simulink model "motor_ctrl_with_PID"  (R2023b)
settings: Solver=FixedStepAuto  StartTime=0.0  StopTime=inf  FixedStep=Ts  RelTol=1e-3
InitFcn:
  | params
  | pin_params
undefined symbols (not defined in the file or in its folder): den_Gd, encoder_scale, J, Kb, KD, Kf, KI, Km, KP, L, num_Gd, R, Vlim, Wref
libraries: arduinolib x12, simulink x6, arduinosensorlib x6
settings Model: SimulationMode=external  ExtModeTrigDuration=2  Creator=SJ  LastModifiedBy=tkdle
settings SolverCC: AutoInsertRateTranBlk=on
settings OptimizationCC: EnhancedBackFolding=on  PassReuseOutputArgsAs=Individual arguments  ZeroExternalMemoryAtStartup=off  ZeroInternalMemoryAtStartup=off  MaxStackSize=64  OptimizeBlockOrder=speed  DifferentSizesBufferReuse=on  OptimizationCustomize=off  EfficientTunableParamExpr=on
settings DebuggingCC: MultiTaskRateTransMsg=warning  ParameterTunabilityLossMsg=error
settings HardwareCC: ProdBitPerInt=16  ProdBitPerPointer=16  ProdBitPerSizeT=16  ProdBitPerPtrDiffT=16  ProdLargestAtomicFloat=None  ProdWordSize=8  ProdHWDeviceType=Atmel->AVR
settings SFSimCC: MATLABDynamicMemAlloc=off
settings RTWCC: Description=Embedded Coder  SystemTargetFile=ert.tlc  HardwareBoard=Arduino Mega 2560  TemplateMakefile=ert_default_tmf  Toolchain=Arduino AVR  BuildConfiguration=Faster Runs
settings CodeAppCC: ForceParamTrailComments=on  IgnoreCustomStorageClasses=off  OperatorAnnotations=on  SimulinkDataObjDesc=on  SFDataObjDesc=on  InsertBlockDesc=on
settings ERTTargetCC: SupportContinuousTime=on  SupportVariableSizeSignals=on  ExtMode=on  ExtModeTransport=3  ExtModeStaticAlloc=on  ExtModeAutomaticAllocSize=off  ExtModeStaticAllocSize=2048  ExtModeMexFile=ext_xcp  ExtModeMexArgs=0 3 921600  ExtModeIntrfLevel=Level2 - Open

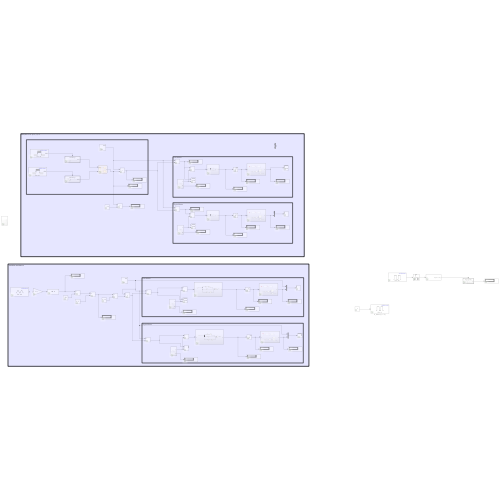
[thumbnail: Simulink's stored preview of the top-level diagram]
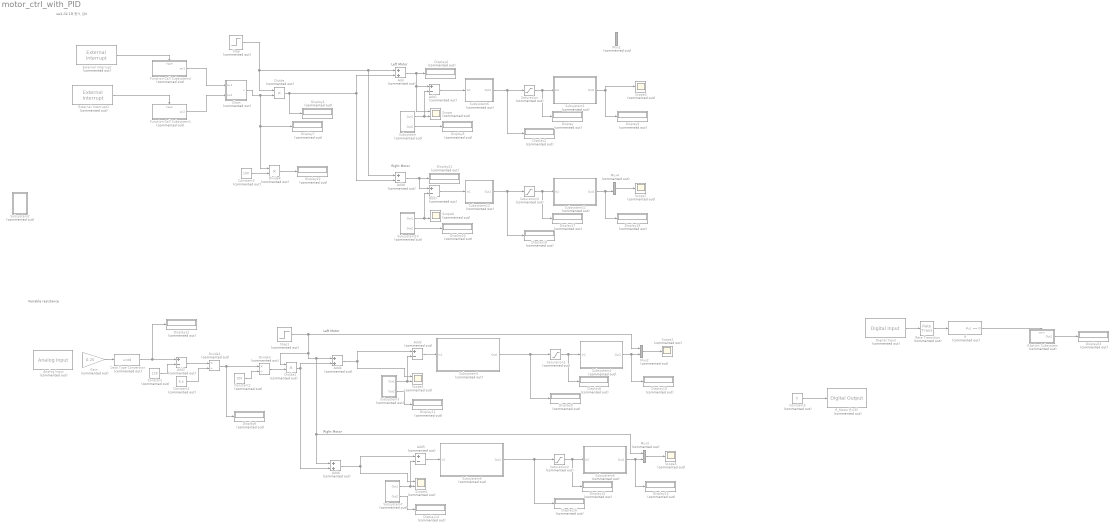
== system motor_ctrl_with_PID ==
  note: Left Motor
  note: Left Motor
  note: Right Motor
  note: Variable resistance
  note: sw1,2로 1퍼 증가, 감소
  note: Right Motor
  Add : Sum  Commented=on
  Add{1..3,5,7..8} (6 alike) : Sum  Commented=on  Inputs=+-
  Add4 : Sum  Commented=on
  Add6 : Sum  Commented=on
  Analog Input : arduinolib/Analog Input  Commented=on  pinNumber=8  ReadResultsOnly=off  ConversionTriggerSource=Software  ExternalTriggerType=uint32( 0 )  OutputDataType=uint16  EnableConversionCompleteNotify=off  EnableOuputStatus=off  SampleTime=-1  blockPlatform=arduino
  Chart : Stateflow chart  Commented=on  TreatAsAtomicUnit=on
  Constant : Constant  Commented=on  Value=128
  Constant1 : Constant  Commented=on  Value=6.4
  Constant2 : Constant  Commented=on  Value=100
  Constant3 : Constant  Commented=on  Value=100
  Constant5 : Constant  Commented=on  Value=0
  Data Type Conversion : DataTypeConversion  Commented=on  OutDataTypeStr=uint8  SaturateOnIntegerOverflow=off  RndMeth=Floor
  Digital Input : arduinolib/Digital Input  Commented=on  pinNumber=20  mode=Default  Direction=input  SampleTime=0.1  blockPlatform=arduino
  Display{,1..23} (24 alike) : Display  Commented=on
  Divide : Product  Commented=on  Inputs=**
  Divide1 : Product  Commented=on  Inputs=*/
  Divide2 : Product  Commented=on  Inputs=**
  Divide3 : Product  Commented=on  Inputs=*/
  Divide4 : Product  Commented=on  Inputs=**
  External Interrupt : arduinolib/External Interrupt  Commented=on  Pin=20  PullUp=off  Mode=FALLING  InterruptSimulationInput=off
  External Interrupt1 : arduinolib/External Interrupt  Commented=on  Pin=21  PullUp=off  Mode=FALLING  InterruptSimulationInput=off
  Function-Call Subsystem1 : Subsystem  Commented=on  TreatAsAtomicUnit=on
  Function-Call Subsystem4 : Subsystem  Commented=on  TreatAsAtomicUnit=on
  Gain : Gain  Commented=on  Gain=0.25
  If : If  Commented=on  IfExpression=u1 == 0  ShowElse=off
  If Action Subsystem : Subsystem  Commented=on  TreatAsAtomicUnit=on
  Mux{1..4} (4 alike) : Mux  Commented=on  Inputs=2
  R_Motor(반시계) : arduinolib/Digital Output  Commented=on  pinNumber=Motor_R_Direction  Direction=output  blockPlatform=arduino
  Rate Transition : RateTransition  Commented=on  OutPortSampleTime=0.5
  Saturation{,1..3} (4 alike) : Saturate  Commented=on  UpperLimit=12  LowerLimit=0
  Scope{,1,4,6} (4 alike) : Scope  Commented=on  NumInputPorts=2
  Scope{2..3,5,7} (4 alike) : Scope  Commented=on
  Step : Step  Commented=on  After=Wref  SampleTime=0
  Step1 : Step  Commented=on  After=Wref  SampleTime=0
  Subsystem : Subsystem  Commented=on
  Subsystem1 : Subsystem  Commented=on
  Subsystem10 : Subsystem  Commented=on
  Subsystem11 : Subsystem  Commented=on
  Subsystem12 : Subsystem  Commented=on
  Subsystem2 : Subsystem  Commented=on
  Subsystem3 : Subsystem  Commented=on
  Subsystem4 : Subsystem  Commented=on
  Subsystem5 : Subsystem  Commented=on
  Subsystem6 : Subsystem  Commented=on
  Subsystem7 : Subsystem  Commented=on
  Subsystem8 : Subsystem  Commented=on
  Subsystem9 : Subsystem  Commented=on
  wires:
  Subsystem/1(Out1) -> Add1/2, Scope/2
  Saturation/1 -> Subsystem1/1(In2), Display/1
  Subsystem1/1(Out1) -> Scope3/1, Display3/1
  External Interrupt/1 -> Function-Call Subsystem4/Trigger
  External Interrupt1/1 -> Function-Call Subsystem1/Trigger
  Function-Call Subsystem4/1(sw1) -> Chart/1(sw1)
  Function-Call Subsystem1/1(sw2) -> Chart/2(sw2)
  Step/1 -> Divide/1, Add8/1, Add/1
  Divide/1 -> Display1/1, Add/2, Add8/2
  Chart/1(n) -> Divide4/1, Display7/1, Divide/2
  Subsystem/2(Out2) -> Display5/1
  Gain/1 -> Data Type Conversion/1
  Step1/1 -> Mux2/1, Add6/1, Mux3/1, Add4/1, Divide2/1
  Data Type Conversion/1 -> Display12/1, Add2/1
  Constant/1 -> Add2/2
  Divide1/1 -> Display6/1, Divide3/1
  Add2/1 -> Divide1/1
  Constant1/1 -> Divide1/2
  Divide2/1 -> Add6/2, Add4/2
  Constant2/1 -> Divide3/2
  Divide3/1 -> Divide2/2
  Add/1 -> Scope/1, Add1/1, Display4/1
  Saturation1/1 -> Subsystem4/1(In2), Display8/1
  Subsystem3/2(Out2) -> Display11/1
  Subsystem3/1(Out1) -> Add3/2, Scope1/2
  Subsystem4/1(Out1) -> Display10/1, Mux2/2
  Mux2/1 -> Scope2/1
  Add4/1 -> Add3/1, Scope1/1
  Subsystem5/1(Out1) -> Display9/1, Saturation1/1
  Add3/1 -> Subsystem5/1(In1)
  Subsystem6/1(Out1) -> Display2/1, Saturation/1
  Add1/1 -> Subsystem6/1(In1)
  Add6/1 -> Add5/1, Scope4/1
  Mux3/1 -> Scope5/1
  Subsystem7/2(Out2) -> Display14/1
  Subsystem8/1(Out1) -> Display13/1, Mux3/2
  Subsystem7/1(Out1) -> Add5/2, Scope4/2
  Add5/1 -> Subsystem9/1(In1)
  Saturation2/1 -> Subsystem8/1(In2), Display15/1
  Subsystem9/1(Out1) -> Display16/1, Saturation2/1
  Add7/1 -> Subsystem12/1(In1)
  Subsystem11/1(Out1) -> Display19/1, Mux4/2
  Saturation3/1 -> Subsystem11/1(In2), Display17/1
  Mux4/1 -> Scope7/1
  Subsystem10/1(Out1) -> Add7/2, Scope6/2
  Subsystem12/1(Out1) -> Display18/1, Saturation3/1
  Subsystem10/2(Out2) -> Display20/1
  Add8/1 -> Add7/1, Display21/1
  Divide4/1 -> Display22/1
  Constant3/1 -> Divide4/2
  Digital Input/1 -> Rate Transition/1
  If/1 -> If Action Subsystem/Action
  If Action Subsystem/1(Out1) -> Display23/1
  Rate Transition/1 -> If/1
  Constant5/1 -> R_Motor(반시계)/1

== system motor_ctrl_with_PID/Function-Call Subsystem1 ==
  function : TriggerPort  TriggerType=function-call  VariantControl=(inherit)
  Add : Sum  Inputs=+-
  Constant : Constant
  Delay : Delay  DelayLength=1
  sw2 : Outport
  wires:
  Add/1 -> Delay/1, sw2/1
  Delay/1 -> Add/2
  Constant/1 -> Add/1

== system motor_ctrl_with_PID/Function-Call Subsystem4 ==
  function : TriggerPort  TriggerType=function-call  VariantControl=(inherit)
  Add : Sum  Inputs=+-
  Constant : Constant
  Delay : Delay  DelayLength=1
  sw1 : Outport
  wires:
  Add/1 -> sw1/1, Delay/1
  Delay/1 -> Add/2
  Constant/1 -> Add/1

== system motor_ctrl_with_PID/If Action Subsystem ==
  Action Port : ActionPort  ActionPortLabel=if(u1 == 0)
  Add : Sum
  Constant : Constant
  Constant1 : Constant  Value=3
  Delay : Delay  DelayLength=1
  Mod : Math  Operator=mod
  Out1 : Outport
  wires:
  Mod/1 -> Delay/1, Out1/1
  Delay/1 -> Add/2
  Constant/1 -> Add/1
  Add/1 -> Mod/1
  Constant1/1 -> Mod/2

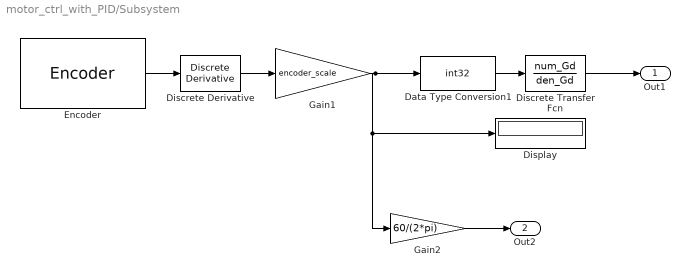
== system motor_ctrl_with_PID/Subsystem ==
  Data Type Conversion1 : DataTypeConversion  OutDataTypeStr=int32  SaturateOnIntegerOverflow=off  RndMeth=Floor
  Discrete Transfer Fcn : DiscreteTransferFcn  Numerator=num_Gd  Denominator=den_Gd
  Discrete Derivative : simulink/Discrete/Discrete Derivative  gainval=1.0  ICPrevScaledInput=0.0  OutMin=[]  OutMax=[]  OutDataType=fixdt(1, 16)  OutScaling=2^-10  DoSatur=off
  Display : Display
  Encoder : arduinosensorlib/Encoder  InputA=18  InputB=19  Mode=No reset  SampleTime=-1
  Gain1 : Gain  Gain=encoder_scale
  Gain2 : Gain  Gain=60/(2*pi)
  Out1 : Outport
  Out2 : Outport  Port=2
  wires:
  Gain1/1 -> Display/1, Gain2/1, Data Type Conversion1/1
  Encoder/1 -> Discrete Derivative/1
  Gain2/1 -> Out2/1
  Data Type Conversion1/1 -> Discrete Transfer Fcn/1
  Discrete Derivative/1 -> Gain1/1
  Discrete Transfer Fcn/1 -> Out1/1

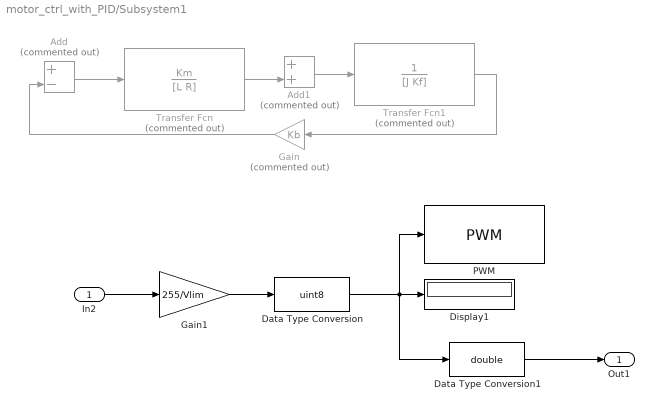
== system motor_ctrl_with_PID/Subsystem1 ==
  In2 : Inport
  Add : Sum  Commented=on  Inputs=+-
  Add1 : Sum  Commented=on
  Data Type Conversion : DataTypeConversion  OutDataTypeStr=uint8  SaturateOnIntegerOverflow=off  RndMeth=Floor
  Data Type Conversion1 : DataTypeConversion  OutDataTypeStr=double  SaturateOnIntegerOverflow=off  RndMeth=Floor
  Display1 : Display
  Gain : Gain  Commented=on  Gain=Kb
  Gain1 : Gain  Gain=255/Vlim
  PWM : arduinolib/PWM  pinNumber=11  frequencyType=Default  desiredFrequency=490.2  achievableFrequency=490.2
  Transfer Fcn : TransferFcn  Commented=on  Numerator=Km  Denominator=[L R]
  Transfer Fcn1 : TransferFcn  Commented=on  Numerator=1  Denominator=[J Kf]
  Out1 : Outport
  wires:
  ? -> Add/1
  ? -> Add1/1
  Add/1 -> Transfer Fcn/1
  Add1/1 -> Transfer Fcn1/1
  Transfer Fcn/1 -> Add1/2
  Gain/1 -> Add/2
  Transfer Fcn1/1 -> Gain/1
  In2/1 -> Gain1/1
  Gain1/1 -> Data Type Conversion/1
  Data Type Conversion1/1 -> Out1/1
  Data Type Conversion/1 -> Data Type Conversion1/1, Display1/1, PWM/1

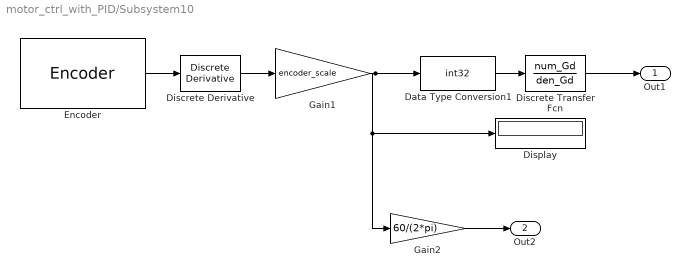
== system motor_ctrl_with_PID/Subsystem10 ==
  Data Type Conversion1 : DataTypeConversion  OutDataTypeStr=int32  SaturateOnIntegerOverflow=off  RndMeth=Floor
  Discrete Transfer Fcn : DiscreteTransferFcn  Numerator=num_Gd  Denominator=den_Gd
  Discrete Derivative : simulink/Discrete/Discrete Derivative  gainval=1.0  ICPrevScaledInput=0.0  OutMin=[]  OutMax=[]  OutDataType=fixdt(1, 16)  OutScaling=2^-10  DoSatur=off
  Display : Display
  Encoder : arduinosensorlib/Encoder  InputA=20  InputB=21  Mode=No reset  SampleTime=-1
  Gain1 : Gain  Gain=encoder_scale
  Gain2 : Gain  Gain=60/(2*pi)
  Out1 : Outport
  Out2 : Outport  Port=2
  wires:
  Gain1/1 -> Display/1, Gain2/1, Data Type Conversion1/1
  Encoder/1 -> Discrete Derivative/1
  Gain2/1 -> Out2/1
  Data Type Conversion1/1 -> Discrete Transfer Fcn/1
  Discrete Derivative/1 -> Gain1/1
  Discrete Transfer Fcn/1 -> Out1/1

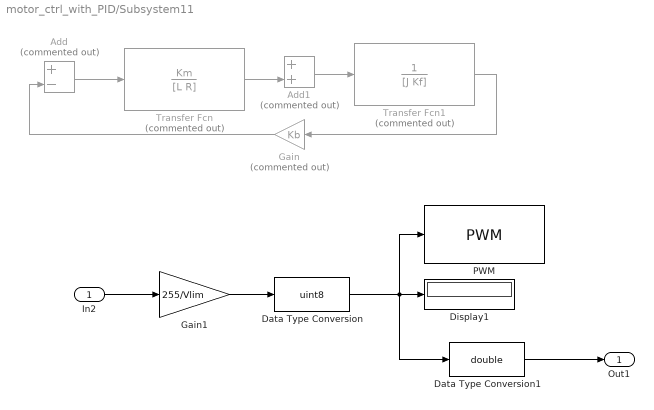
== system motor_ctrl_with_PID/Subsystem11 ==
  In2 : Inport
  Add : Sum  Commented=on  Inputs=+-
  Add1 : Sum  Commented=on
  Data Type Conversion : DataTypeConversion  OutDataTypeStr=uint8  SaturateOnIntegerOverflow=off  RndMeth=Floor
  Data Type Conversion1 : DataTypeConversion  OutDataTypeStr=double  SaturateOnIntegerOverflow=off  RndMeth=Floor
  Display1 : Display
  Gain : Gain  Commented=on  Gain=Kb
  Gain1 : Gain  Gain=255/Vlim
  PWM : arduinolib/PWM  pinNumber=11  frequencyType=Default  desiredFrequency=490.2  achievableFrequency=490.2
  Transfer Fcn : TransferFcn  Commented=on  Numerator=Km  Denominator=[L R]
  Transfer Fcn1 : TransferFcn  Commented=on  Numerator=1  Denominator=[J Kf]
  Out1 : Outport
  wires:
  ? -> Add/1
  ? -> Add1/1
  Add/1 -> Transfer Fcn/1
  Add1/1 -> Transfer Fcn1/1
  Transfer Fcn/1 -> Add1/2
  Gain/1 -> Add/2
  Transfer Fcn1/1 -> Gain/1
  In2/1 -> Gain1/1
  Gain1/1 -> Data Type Conversion/1
  Data Type Conversion1/1 -> Out1/1
  Data Type Conversion/1 -> Data Type Conversion1/1, Display1/1, PWM/1

== system motor_ctrl_with_PID/Subsystem12 ==
  In1 : Inport
  Derivative1 : Derivative  Commented=on
  Gain4 : Gain  Commented=on  Gain=KI
  Gain5 : Gain  Commented=on  Gain=KP
  Gain6 : Gain  Commented=on  Gain=KD
  Integrator1 : Integrator  Commented=on
  Subtract1 : Sum  Commented=on  Inputs=+++
  Out1 : Outport
  wires:
  Derivative1/1 -> Subtract1/3
  Gain4/1 -> Integrator1/1
  Integrator1/1 -> Subtract1/1
  Gain6/1 -> Derivative1/1
  Subtract1/1 -> Out1/1
  In1/1 -> Gain5/1, Gain6/1, Gain4/1
  Gain5/1 -> Subtract1/2

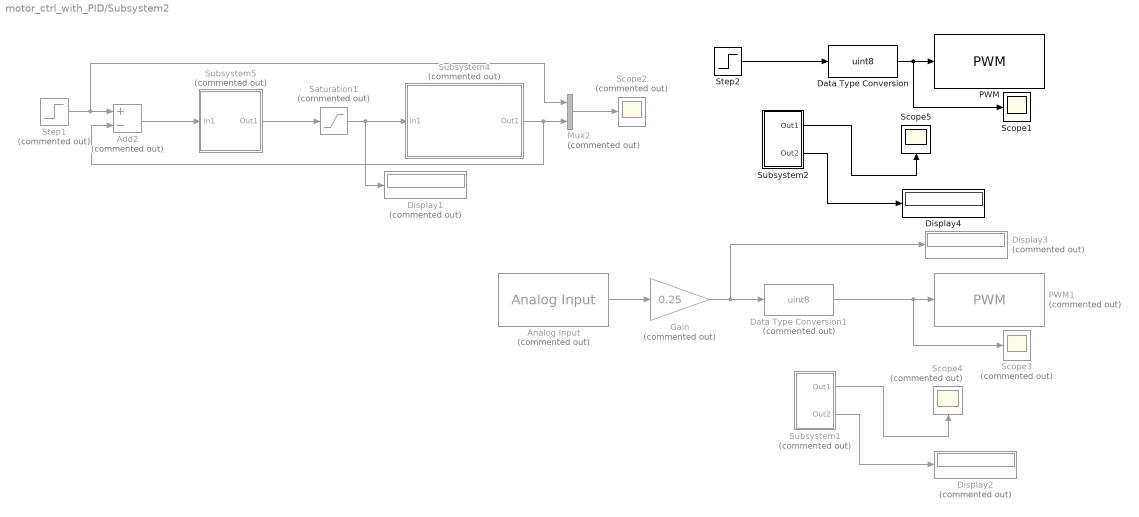
== system motor_ctrl_with_PID/Subsystem2 ==
  Add2 : Sum  Commented=on  Inputs=+-
  Analog Input : arduinolib/Analog Input  Commented=on  pinNumber=8  ReadResultsOnly=off  ConversionTriggerSource=Software  ExternalTriggerType=uint32( 0 )  OutputDataType=uint16  EnableConversionCompleteNotify=off  EnableOuputStatus=off  SampleTime=-1  blockPlatform=arduino
  Data Type Conversion : DataTypeConversion  OutDataTypeStr=uint8  SaturateOnIntegerOverflow=off  RndMeth=Floor
  Data Type Conversion1 : DataTypeConversion  Commented=on  OutDataTypeStr=uint8  SaturateOnIntegerOverflow=off  RndMeth=Floor
  Display1 : Display  Commented=on
  Display2 : Display  Commented=on
  Display3 : Display  Commented=on
  Display4 : Display
  Gain : Gain  Commented=on  Gain=0.25
  Mux2 : Mux  Commented=on  Inputs=2
  PWM : arduinolib/PWM  pinNumber=11  frequencyType=Default  desiredFrequency=490.2  achievableFrequency=490.2
  PWM1 : arduinolib/PWM  Commented=on  pinNumber=11  frequencyType=Default  desiredFrequency=490.2  achievableFrequency=490.2
  Saturation1 : Saturate  Commented=on  UpperLimit=Vlim  LowerLimit=0
  Scope1 : Scope
  Scope2 : Scope  Commented=on
  Scope3 : Scope  Commented=on
  Scope4 : Scope  Commented=on
  Scope5 : Scope
  Step1 : Step  Commented=on  After=Wref  SampleTime=0
  Step2 : Step  After=Wref  SampleTime=0
  Subsystem1 : Subsystem  Commented=on
  Subsystem2 : Subsystem
  Subsystem4 : Subsystem  Commented=on
  Subsystem5 : Subsystem  Commented=on
  wires:
  Data Type Conversion/1 -> Scope1/1, PWM/1
  Add2/1 -> Subsystem5/1(In1)
  Saturation1/1 -> Subsystem4/1(In1), Display1/1
  Mux2/1 -> Scope2/1
  Subsystem4/1(Out1) -> Add2/2, Mux2/2
  Step2/1 -> Data Type Conversion/1
  Subsystem5/1(Out1) -> Saturation1/1
  Step1/1 -> Mux2/1, Add2/1
  Subsystem1/1(Out1) -> Scope4/1
  Gain/1 -> Display3/1, Data Type Conversion1/1
  Data Type Conversion1/1 -> Scope3/1, PWM1/1
  Analog Input/1 -> Gain/1
  Subsystem1/2(Out2) -> Display2/1
  Subsystem2/1(Out1) -> Scope5/1
  Subsystem2/2(Out2) -> Display4/1

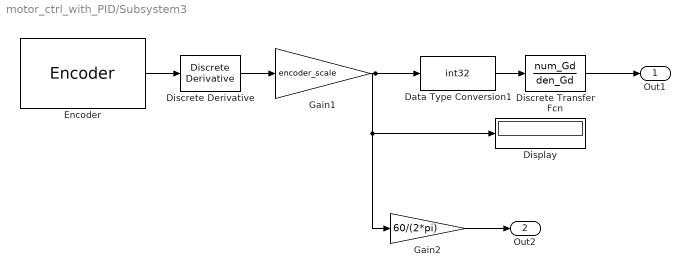
== system motor_ctrl_with_PID/Subsystem3 ==
  Data Type Conversion1 : DataTypeConversion  OutDataTypeStr=int32  SaturateOnIntegerOverflow=off  RndMeth=Floor
  Discrete Transfer Fcn : DiscreteTransferFcn  Numerator=num_Gd  Denominator=den_Gd
  Discrete Derivative : simulink/Discrete/Discrete Derivative  gainval=1.0  ICPrevScaledInput=0.0  OutMin=[]  OutMax=[]  OutDataType=fixdt(1, 16)  OutScaling=2^-10  DoSatur=off
  Display : Display
  Encoder : arduinosensorlib/Encoder  InputA=18  InputB=19  Mode=No reset  SampleTime=-1
  Gain1 : Gain  Gain=encoder_scale
  Gain2 : Gain  Gain=60/(2*pi)
  Out1 : Outport
  Out2 : Outport  Port=2
  wires:
  Gain1/1 -> Display/1, Gain2/1, Data Type Conversion1/1
  Encoder/1 -> Discrete Derivative/1
  Gain2/1 -> Out2/1
  Data Type Conversion1/1 -> Discrete Transfer Fcn/1
  Discrete Derivative/1 -> Gain1/1
  Discrete Transfer Fcn/1 -> Out1/1

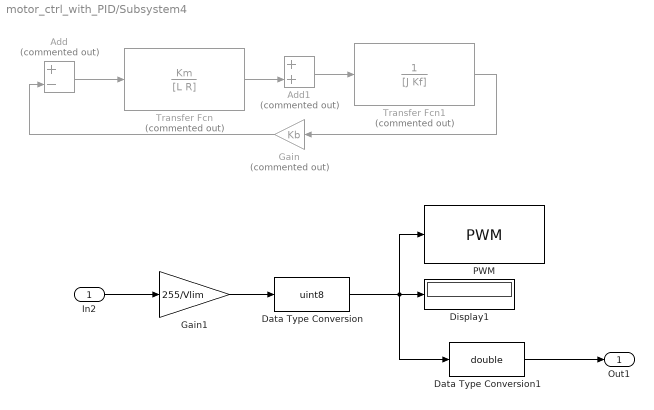
== system motor_ctrl_with_PID/Subsystem4 ==
  In2 : Inport
  Add : Sum  Commented=on  Inputs=+-
  Add1 : Sum  Commented=on
  Data Type Conversion : DataTypeConversion  OutDataTypeStr=uint8  SaturateOnIntegerOverflow=off  RndMeth=Floor
  Data Type Conversion1 : DataTypeConversion  OutDataTypeStr=double  SaturateOnIntegerOverflow=off  RndMeth=Floor
  Display1 : Display
  Gain : Gain  Commented=on  Gain=Kb
  Gain1 : Gain  Gain=255/Vlim
  PWM : arduinolib/PWM  pinNumber=11  frequencyType=Default  desiredFrequency=490.2  achievableFrequency=490.2
  Transfer Fcn : TransferFcn  Commented=on  Numerator=Km  Denominator=[L R]
  Transfer Fcn1 : TransferFcn  Commented=on  Numerator=1  Denominator=[J Kf]
  Out1 : Outport
  wires:
  ? -> Add/1
  ? -> Add1/1
  Add/1 -> Transfer Fcn/1
  Add1/1 -> Transfer Fcn1/1
  Transfer Fcn/1 -> Add1/2
  Gain/1 -> Add/2
  Transfer Fcn1/1 -> Gain/1
  In2/1 -> Gain1/1
  Gain1/1 -> Data Type Conversion/1
  Data Type Conversion1/1 -> Out1/1
  Data Type Conversion/1 -> Data Type Conversion1/1, Display1/1, PWM/1

== system motor_ctrl_with_PID/Subsystem5 ==
  In1 : Inport
  Derivative2 : Derivative
  Gain1 : Gain  Gain=KI
  Gain2 : Gain  Gain=KP
  Gain3 : Gain  Gain=KD
  Integrator2 : Integrator
  Subtract2 : Sum  Inputs=+++
  Out1 : Outport
  wires:
  Gain1/1 -> Integrator2/1
  Gain2/1 -> Subtract2/2
  Integrator2/1 -> Subtract2/1
  In1/1 -> Gain2/1, Gain3/1, Gain1/1
  Derivative2/1 -> Subtract2/3
  Gain3/1 -> Derivative2/1
  Subtract2/1 -> Out1/1

== system motor_ctrl_with_PID/Subsystem6 ==
  In1 : Inport
  Derivative1 : Derivative
  Gain4 : Gain  Gain=KI
  Gain5 : Gain  Gain=KP
  Gain6 : Gain  Gain=KD
  Integrator1 : Integrator
  Subtract1 : Sum  Inputs=+++
  Out1 : Outport
  wires:
  Derivative1/1 -> Subtract1/3
  Gain4/1 -> Integrator1/1
  Integrator1/1 -> Subtract1/1
  Gain6/1 -> Derivative1/1
  Subtract1/1 -> Out1/1
  In1/1 -> Gain5/1, Gain6/1, Gain4/1
  Gain5/1 -> Subtract1/2

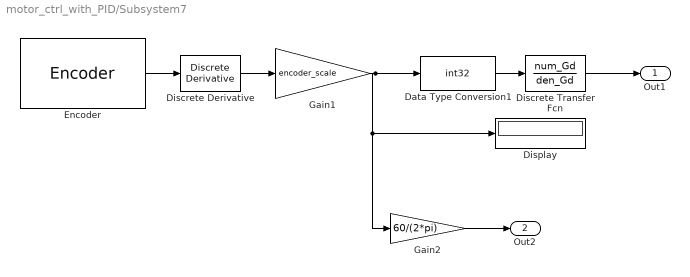
== system motor_ctrl_with_PID/Subsystem7 ==
  Data Type Conversion1 : DataTypeConversion  OutDataTypeStr=int32  SaturateOnIntegerOverflow=off  RndMeth=Floor
  Discrete Transfer Fcn : DiscreteTransferFcn  Numerator=num_Gd  Denominator=den_Gd
  Discrete Derivative : simulink/Discrete/Discrete Derivative  gainval=1.0  ICPrevScaledInput=0.0  OutMin=[]  OutMax=[]  OutDataType=fixdt(1, 16)  OutScaling=2^-10  DoSatur=off
  Display : Display
  Encoder : arduinosensorlib/Encoder  InputA=20  InputB=21  Mode=No reset  SampleTime=-1
  Gain1 : Gain  Gain=encoder_scale
  Gain2 : Gain  Gain=60/(2*pi)
  Out1 : Outport
  Out2 : Outport  Port=2
  wires:
  Gain1/1 -> Display/1, Gain2/1, Data Type Conversion1/1
  Encoder/1 -> Discrete Derivative/1
  Gain2/1 -> Out2/1
  Data Type Conversion1/1 -> Discrete Transfer Fcn/1
  Discrete Derivative/1 -> Gain1/1
  Discrete Transfer Fcn/1 -> Out1/1

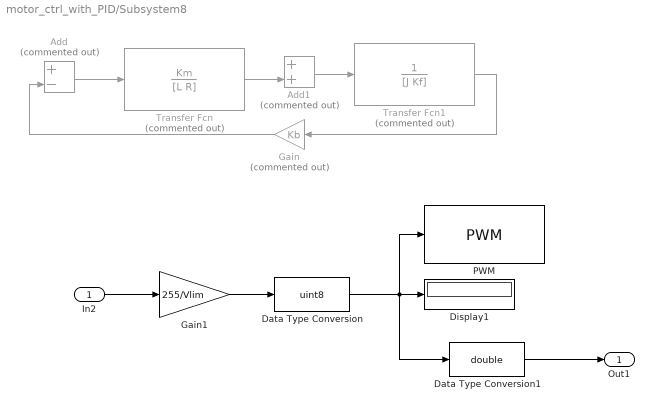
== system motor_ctrl_with_PID/Subsystem8 ==
  In2 : Inport
  Add : Sum  Commented=on  Inputs=+-
  Add1 : Sum  Commented=on
  Data Type Conversion : DataTypeConversion  OutDataTypeStr=uint8  SaturateOnIntegerOverflow=off  RndMeth=Floor
  Data Type Conversion1 : DataTypeConversion  OutDataTypeStr=double  SaturateOnIntegerOverflow=off  RndMeth=Floor
  Display1 : Display
  Gain : Gain  Commented=on  Gain=Kb
  Gain1 : Gain  Gain=255/Vlim
  PWM : arduinolib/PWM  pinNumber=3  frequencyType=Default  desiredFrequency=490.2  achievableFrequency=490.2
  Transfer Fcn : TransferFcn  Commented=on  Numerator=Km  Denominator=[L R]
  Transfer Fcn1 : TransferFcn  Commented=on  Numerator=1  Denominator=[J Kf]
  Out1 : Outport
  wires:
  ? -> Add/1
  ? -> Add1/1
  Add/1 -> Transfer Fcn/1
  Add1/1 -> Transfer Fcn1/1
  Transfer Fcn/1 -> Add1/2
  Gain/1 -> Add/2
  Transfer Fcn1/1 -> Gain/1
  In2/1 -> Gain1/1
  Gain1/1 -> Data Type Conversion/1
  Data Type Conversion1/1 -> Out1/1
  Data Type Conversion/1 -> Data Type Conversion1/1, Display1/1, PWM/1

== system motor_ctrl_with_PID/Subsystem9 ==
  In1 : Inport
  Derivative2 : Derivative
  Gain1 : Gain  Gain=KI
  Gain2 : Gain  Gain=KP
  Gain3 : Gain  Gain=KD
  Integrator2 : Integrator
  Subtract2 : Sum  Inputs=+++
  Out1 : Outport
  wires:
  Gain1/1 -> Integrator2/1
  Gain2/1 -> Subtract2/2
  Integrator2/1 -> Subtract2/1
  In1/1 -> Gain2/1, Gain3/1, Gain1/1
  Derivative2/1 -> Subtract2/3
  Gain3/1 -> Derivative2/1
  Subtract2/1 -> Out1/1

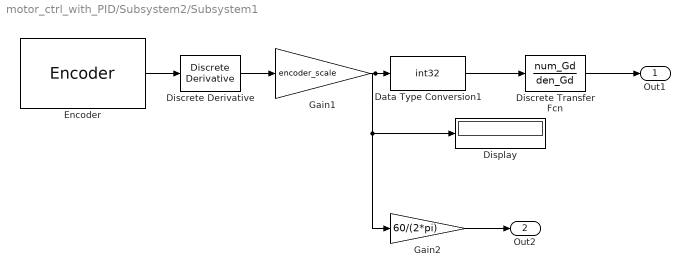
== system motor_ctrl_with_PID/Subsystem2/Subsystem1 ==
  Data Type Conversion1 : DataTypeConversion  OutDataTypeStr=int32  SaturateOnIntegerOverflow=off  RndMeth=Floor
  Discrete Transfer Fcn : DiscreteTransferFcn  Numerator=num_Gd  Denominator=den_Gd
  Discrete Derivative : simulink/Discrete/Discrete Derivative  gainval=1.0  ICPrevScaledInput=0.0  OutMin=[]  OutMax=[]  OutDataType=fixdt(1, 16)  OutScaling=2^-10  DoSatur=off
  Display : Display
  Encoder : arduinosensorlib/Encoder  InputA=18  InputB=19  Mode=No reset  SampleTime=-1
  Gain1 : Gain  Gain=encoder_scale
  Gain2 : Gain  Gain=60/(2*pi)
  Out1 : Outport
  Out2 : Outport  Port=2
  wires:
  Gain1/1 -> Display/1, Gain2/1, Data Type Conversion1/1
  Encoder/1 -> Discrete Derivative/1
  Gain2/1 -> Out2/1
  Data Type Conversion1/1 -> Discrete Transfer Fcn/1
  Discrete Derivative/1 -> Gain1/1
  Discrete Transfer Fcn/1 -> Out1/1

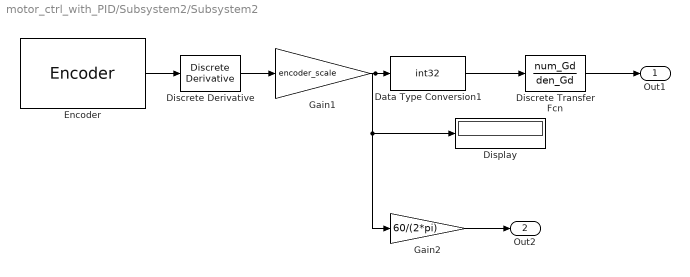
== system motor_ctrl_with_PID/Subsystem2/Subsystem2 ==
  Data Type Conversion1 : DataTypeConversion  OutDataTypeStr=int32  SaturateOnIntegerOverflow=off  RndMeth=Floor
  Discrete Transfer Fcn : DiscreteTransferFcn  Numerator=num_Gd  Denominator=den_Gd
  Discrete Derivative : simulink/Discrete/Discrete Derivative  gainval=1.0  ICPrevScaledInput=0.0  OutMin=[]  OutMax=[]  OutDataType=fixdt(1, 16)  OutScaling=2^-10  DoSatur=off
  Display : Display
  Encoder : arduinosensorlib/Encoder  InputA=18  InputB=19  Mode=No reset  SampleTime=-1
  Gain1 : Gain  Gain=encoder_scale
  Gain2 : Gain  Gain=60/(2*pi)
  Out1 : Outport
  Out2 : Outport  Port=2
  wires:
  Gain1/1 -> Display/1, Gain2/1, Data Type Conversion1/1
  Encoder/1 -> Discrete Derivative/1
  Gain2/1 -> Out2/1
  Data Type Conversion1/1 -> Discrete Transfer Fcn/1
  Discrete Derivative/1 -> Gain1/1
  Discrete Transfer Fcn/1 -> Out1/1

== system motor_ctrl_with_PID/Subsystem2/Subsystem4 ==
  In1 : Inport
  Add : Sum  Inputs=+-
  Add1 : Sum
  Gain : Gain  Gain=Kb
  Transfer Fcn : TransferFcn  Numerator=Km  Denominator=[L R]
  Transfer Fcn1 : TransferFcn  Numerator=1  Denominator=[J Kf]
  Out1 : Outport
  wires:
  In1/1 -> Add/1
  ? -> Add1/1
  Add/1 -> Transfer Fcn/1
  Add1/1 -> Transfer Fcn1/1
  Transfer Fcn/1 -> Add1/2
  Gain/1 -> Add/2
  Transfer Fcn1/1 -> Gain/1, Out1/1

== system motor_ctrl_with_PID/Subsystem2/Subsystem5 ==
  In1 : Inport
  Derivative1 : Derivative
  Gain4 : Gain  Gain=KI
  Gain5 : Gain  Gain=KP
  Gain6 : Gain  Gain=KD
  Integrator1 : Integrator
  Subtract1 : Sum  Inputs=+++
  Out1 : Outport
  wires:
  Subtract1/1 -> Out1/1
  In1/1 -> Gain5/1, Gain6/1, Gain4/1
  Integrator1/1 -> Subtract1/1
  Derivative1/1 -> Subtract1/3
  Gain6/1 -> Derivative1/1
  Gain5/1 -> Subtract1/2
  Gain4/1 -> Integrator1/1

== stateflow chart motor_ctrl_with_PID/Chart ==
  state AccOff
    en: state=state+1;
    v1=sw1;
    v2=sw2;
    n=state/100
    du:
  state AccStandby
    en: state=state+1;
    v1=sw1;
    v2=sw2;
    n=state/100
    du:
  state AccOn1
    en: state=state-1;
    v1=sw1;
    v2=sw2;
    n=state/100
    du:
  state AccOn
    en: state=state-1;
    v1=sw1;
    v2=sw2;
    n=state/100
    du:
  (default) -> AccOff : {state=-1}
  AccOff -> AccStandby [order 1] : [v1~=sw1]
  AccStandby -> AccOff [order 1] : [v1~=sw1]
  AccOff -> AccOn [order 2] : [v2~=sw2]
  AccOn -> AccOff [order 2] : [v1~=sw1]
  AccOn1 -> AccStandby [order 1] : [v1~=sw1]
  AccStandby -> AccOn1 [order 2] : [v2~=sw2]
  AccOn1 -> AccOn [order 2] : [v2~=sw2]
  AccOn -> AccOn1 [order 1] : [v2~=sw2]
  data: sw1 input; v1 local; v2 local; sw2 input; n output; state local
